simulink model "quadrocopter_simulink"  (R2019a)
settings: Solver=VariableStepAuto  StartTime=0.0  StopTime=100  MaxStep=0.01  RelTol=1e-3
values from neighbouring files (symbols this model uses):
  g = 9.8    [data.m]
  Kd = 5e3    (= 5000)    [data.m]
  Kp = 3.3e5    (= 330000)    [data.m]
  m = 2    [data.m]
  w0 = m*g/(4*b)    (= 0.98)    [data.m]
  zend = 200    [data.m]
settings Model: Creator=Rike Voltz  LastModifiedBy=Rike Voltz

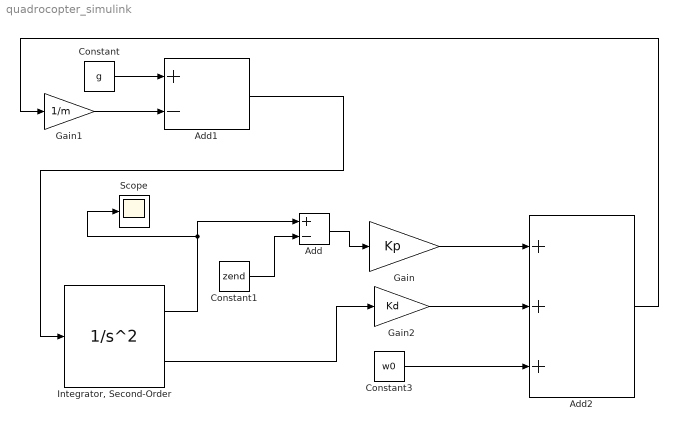
== system quadrocopter_simulink ==
  Add : Sum  Inputs=+-
  Add1 : Sum  Inputs=+-
  Add2 : Sum  Inputs=+++
  Constant : Constant  Value=g
  Constant1 : Constant  Value=zend
  Constant3 : Constant  Value=w0
  Gain : Gain  Gain=Kp
  Gain1 : Gain  Gain=1/m
  Gain2 : Gain  Gain=Kd
  "Integrator, Second-Order" : SecondOrderIntegrator
  Scope : Scope
  wires:
  Constant/1 -> Add1/1
  "Integrator, Second-Order"/1 -> Add/1, Scope/1
  Add1/1 -> "Integrator, Second-Order"/1
  Gain1/1 -> Add1/2
  Gain/1 -> Add2/1
  Constant3/1 -> Add2/3
  Add2/1 -> Gain1/1
  Add/1 -> Gain/1
  Gain2/1 -> Add2/2
  "Integrator, Second-Order"/2 -> Gain2/1
  Constant1/1 -> Add/2
